simulink model "Pacemaker"  (R2020a)
settings: Solver=FixedStepAuto  StartTime=0.0  StopTime=10.0  FixedStep=1e-3  RelTol=1e-3  EnableMultiTasking=on
undefined symbols (not defined in the file): ATR_CMP_REF_PWM, ATR_GND_CTRL, ATR_PACE_CTRL, FRONTEND_CTRL, PACE_CHARGE_CTRL, PACE_GND_CTRL, PACING_REF_PWM, VENT_CMP_REF_PWM, VENT_GND_CTRL, VENT_PACE_CTRL, Z_ATR_CTRL, Z_VENT_CTRL
libraries: frdmk64flib x1
settings Model: ExtModeTrigDuration=5  Creator=Tim_G  LastModifiedBy=Tim_G
settings OptimizationCC: EnhancedBackFolding=on  PassReuseOutputArgsAs=Individual arguments  ZeroExternalMemoryAtStartup=off  ZeroInternalMemoryAtStartup=off  MaxStackSize=64  OptimizeBlockOrder=speed  DifferentSizesBufferReuse=on  OptimizationCustomize=off  EfficientTunableParamExpr=on
settings DebuggingCC: ParameterTunabilityLossMsg=error
settings HardwareCC: ProdBitPerPointer=32  ProdBitPerSizeT=32  ProdBitPerPtrDiffT=32  ProdLargestAtomicInteger=Long  ProdLargestAtomicFloat=Double  ProdWordSize=32  ProdHWDeviceType=ARM Compatible->ARM Cortex
settings SFSimCC: MATLABDynamicMemAlloc=off
settings RTWCC: SystemTargetFile=ert.tlc  HardwareBoard=NXP FRDM-K64F  TemplateMakefile=ert_default_tmf  Toolchain=GNU Tools for ARM Embedded Processors
settings CodeAppCC: ForceParamTrailComments=on  IgnoreCustomStorageClasses=off  OperatorAnnotations=on  SimulinkDataObjDesc=on  SFDataObjDesc=on  InsertBlockDesc=on

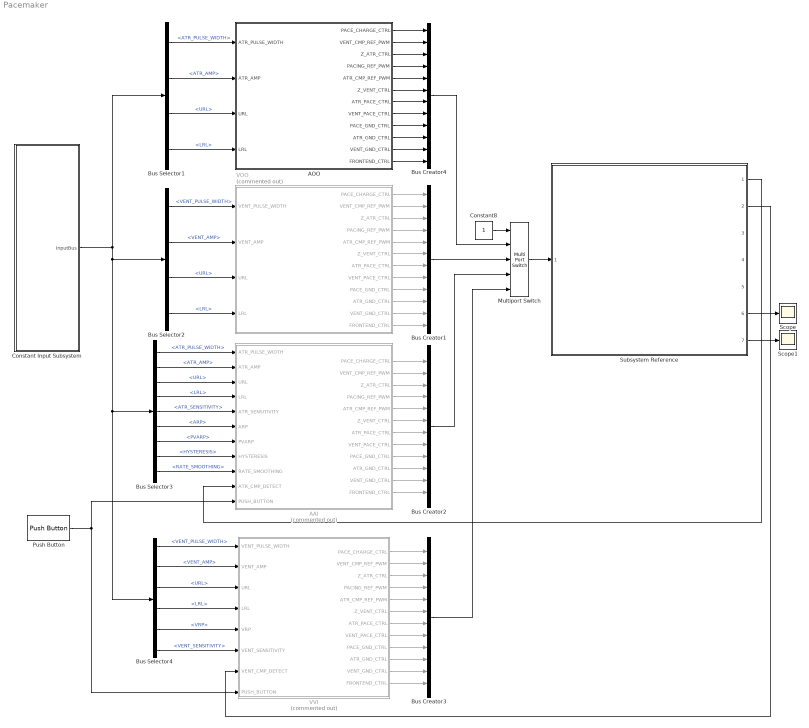
== system Pacemaker ==
  AAI : Stateflow chart  Commented=on  TreatAsAtomicUnit=on
      settings: PortSchema="{\"entries\":[{\"content\":{\"sides\":[{\"content\":{\"connectorIds\":[\"In1\",\"In2\",\"In3\",\"In4\",\"In6\",\"In5\",\"In8\",\"In9\",\"In10\",\"In7\",\"In11\"]},\"type\":\"ConnectorPlacement.EquallySpacedRectSide\",\"uuid\":\"15e17ad8-b4d5-4618-94ec-328f447b5375\"},{\"content\":{\"connectorIds\":[\"Out1\",\"Out2\",\"Out3\",\"Out4\",\"Out5\",\"Out6\",\"Out7\",\"Out8\",\"Out9\",\"Out10\",\"Out11\",\"Out12\"],\"side\":\"RIGHT\"},\"type\":\"ConnectorPlacement.EquallySpacedRectSide\",\"uuid\":\"1d62d0c4-23d6-4fac-9825-8cf7a4b74954\"},{\"content\":{\"connectorIds\":[],\"side\":\"TOP\"},\"type\":\"ConnectorPlacement.EquallySpacedRectSide\",\"uuid\":\"6d7cbaed-215f-4550-bcf7-2324ed1fe24a\"}]},\"type\":\"ConnectorPlacement.EquallySpacedConnector\",\"uuid\":\"41d78d22-c4a1-401b-9b90-f67359ce816a\"}],\"packageUris\":[\"http://schema.mathworks.com/mf0/Connector/19700101\"],\"version\":\"1.0\"}"
  AOO : Stateflow chart  TreatAsAtomicUnit=on
  Bus Creator{1..4} (4 alike) : BusCreator  Inputs=PACE_CHARGE_CTRL,VENT_CMP_REF_PWM,Z_ATR_CTRL,PACING_REF_PWM,ATR_CMP_REF_PWM,Z_VENT_CTRL,ATR_PACE_CTRL,VENT_PACE_CTRL,PACE_GND_CTRL,ATR_GND_CTRL,VENT_GND_CTRL,FRONTEND_CTRL
  Bus Selector1 : BusSelector  OutputSignals=ATR_PULSE_WIDTH,ATR_AMP,URL,LRL
  Bus Selector2 : BusSelector  OutputSignals=VENT_PULSE_WIDTH,VENT_AMP,URL,LRL
  Bus Selector3 : BusSelector  OutputSignals=ATR_PULSE_WIDTH,ATR_AMP,URL,LRL,ATR_SENSITIVITY,ARP,PVARP,HYSTERESIS,RATE_SMOOTHING
  Bus Selector4 : BusSelector  OutputSignals=VENT_PULSE_WIDTH,VENT_AMP,URL,LRL,VRP,VENT_SENSITIVITY
  Constant Input Subsystem : Subsystem
  Constant8 : Constant
  Multiport Switch : MultiPortSwitch  Inputs=4
  Push Button : frdmk64flib/Push Button  Whichswitch=SW2  SampleTime1=-1
  Scope : Scope
  Scope1 : Scope
  Subsystem Reference : Subsystem  ReferencedSubsystem=k64f_hardware_subsystem
  VOO : Stateflow chart  Commented=on  TreatAsAtomicUnit=on
  VVI : Stateflow chart  Commented=on  TreatAsAtomicUnit=on
  wires:
  AAI/3(Z_ATR_CTRL) -> Bus Creator2/3
  AAI/10(ATR_GND_CTRL) -> Bus Creator2/10
  AAI/11(VENT_GND_CTRL) -> Bus Creator2/11
  AAI/12(FRONTEND_CTRL) -> Bus Creator2/12
  Bus Creator2/1 -> Multiport Switch/4
  AAI/5(ATR_CMP_REF_PWM) -> Bus Creator2/5
  AAI/6(Z_VENT_CTRL) -> Bus Creator2/6
  AAI/4(PACING_REF_PWM) -> Bus Creator2/4
  AAI/9(PACE_GND_CTRL) -> Bus Creator2/9
  AAI/8(VENT_PACE_CTRL) -> Bus Creator2/8
  AAI/7(ATR_PACE_CTRL) -> Bus Creator2/7
  Bus Creator1/1 -> Multiport Switch/3
  Subsystem Reference/2 -> VVI/7(VENT_CMP_DETECT)
  AAI/1(PACE_CHARGE_CTRL) -> Bus Creator2/1
  Subsystem Reference/1 -> AAI/7(ATR_CMP_DETECT)
  Bus Creator4/1 -> Multiport Switch/2
  Constant8/1 -> Multiport Switch/1
  VVI/1(PACE_CHARGE_CTRL) -> Bus Creator3/1
  VVI/2(VENT_CMP_REF_PWM) -> Bus Creator3/2
  VVI/3(Z_ATR_CTRL) -> Bus Creator3/3
  VVI/4(PACING_REF_PWM) -> Bus Creator3/4
  VVI/6(Z_VENT_CTRL) -> Bus Creator3/6
  VVI/7(ATR_PACE_CTRL) -> Bus Creator3/7
  VVI/8(VENT_PACE_CTRL) -> Bus Creator3/8
  VVI/9(PACE_GND_CTRL) -> Bus Creator3/9
  VVI/10(ATR_GND_CTRL) -> Bus Creator3/10
  VVI/11(VENT_GND_CTRL) -> Bus Creator3/11
  VVI/12(FRONTEND_CTRL) -> Bus Creator3/12
  Bus Creator3/1 -> Multiport Switch/5
  Bus Selector1/1 -> AOO/1(ATR_PULSE_WIDTH)  "<ATR_PULSE_WIDTH>"
  Bus Selector1/2 -> AOO/2(ATR_AMP)  "<ATR_AMP>"
  Bus Selector1/3 -> AOO/3(URL)  "<URL>"
  Bus Selector1/4 -> AOO/4(LRL)  "<LRL>"
  Bus Selector3/1 -> AAI/1(ATR_PULSE_WIDTH)  "<ATR_PULSE_WIDTH>"
  Bus Selector3/2 -> AAI/2(ATR_AMP)  "<ATR_AMP>"
  Bus Selector3/3 -> AAI/3(URL)  "<URL>"
  Bus Selector3/4 -> AAI/4(LRL)  "<LRL>"
  Bus Selector3/7 -> AAI/8(PVARP)  "<PVARP>"
  Bus Selector3/8 -> AAI/9(HYSTERESIS)  "<HYSTERESIS>"
  Bus Selector3/9 -> AAI/10(RATE_SMOOTHING)  "<RATE_SMOOTHING>"
  Bus Selector3/5 -> AAI/6(ATR_SENSITIVITY)  "<ATR_SENSITIVITY>"
  Bus Selector3/6 -> AAI/5(ARP)  "<ARP>"
  Bus Selector4/1 -> VVI/1(VENT_PULSE_WIDTH)  "<VENT_PULSE_WIDTH>"
  Bus Selector4/2 -> VVI/2(VENT_AMP)  "<VENT_AMP>"
  Bus Selector4/3 -> VVI/3(URL)  "<URL>"
  Bus Selector4/4 -> VVI/4(LRL)  "<LRL>"
  Bus Selector4/5 -> VVI/5(VRP)  "<VRP>"
  Bus Selector4/6 -> VVI/6(VENT_SENSITIVITY)  "<VENT_SENSITIVITY>"
  Constant Input Subsystem/1(InputBus) -> Bus Selector2/1, Bus Selector4/1, Bus Selector3/1, Bus Selector1/1
  Push Button/1 -> VVI/8(PUSH_BUTTON), AAI/11(PUSH_BUTTON)
  AOO/1(PACE_CHARGE_CTRL) -> Bus Creator4/1
  AOO/2(VENT_CMP_REF_PWM) -> Bus Creator4/2
  AOO/3(Z_ATR_CTRL) -> Bus Creator4/3
  AOO/4(PACING_REF_PWM) -> Bus Creator4/4
  AOO/5(ATR_CMP_REF_PWM) -> Bus Creator4/5
  AOO/6(Z_VENT_CTRL) -> Bus Creator4/6
  AOO/7(ATR_PACE_CTRL) -> Bus Creator4/7
  AOO/8(VENT_PACE_CTRL) -> Bus Creator4/8
  AOO/9(PACE_GND_CTRL) -> Bus Creator4/9
  AOO/10(ATR_GND_CTRL) -> Bus Creator4/10
  AOO/11(VENT_GND_CTRL) -> Bus Creator4/11
  AOO/12(FRONTEND_CTRL) -> Bus Creator4/12
  VOO/1(PACE_CHARGE_CTRL) -> Bus Creator1/1
  VOO/2(VENT_CMP_REF_PWM) -> Bus Creator1/2
  VOO/3(Z_ATR_CTRL) -> Bus Creator1/3
  VOO/4(PACING_REF_PWM) -> Bus Creator1/4
  VOO/5(ATR_CMP_REF_PWM) -> Bus Creator1/5
  VOO/6(Z_VENT_CTRL) -> Bus Creator1/6
  VOO/7(ATR_PACE_CTRL) -> Bus Creator1/7
  VOO/8(VENT_PACE_CTRL) -> Bus Creator1/8
  VOO/9(PACE_GND_CTRL) -> Bus Creator1/9
  VOO/10(ATR_GND_CTRL) -> Bus Creator1/10
  VOO/11(VENT_GND_CTRL) -> Bus Creator1/11
  VOO/12(FRONTEND_CTRL) -> Bus Creator1/12
  AAI/2(VENT_CMP_REF_PWM) -> Bus Creator2/2
  VVI/5(ATR_CMP_REF_PWM) -> Bus Creator3/5
  Bus Selector2/1 -> VOO/1(VENT_PULSE_WIDTH)  "<VENT_PULSE_WIDTH>"
  Bus Selector2/2 -> VOO/2(VENT_AMP)  "<VENT_AMP>"
  Bus Selector2/3 -> VOO/3(URL)  "<URL>"
  Bus Selector2/4 -> VOO/4(LRL)  "<LRL>"
  Multiport Switch/1 -> Subsystem Reference/1
  Subsystem Reference/7 -> Scope1/1
  Subsystem Reference/6 -> Scope/1

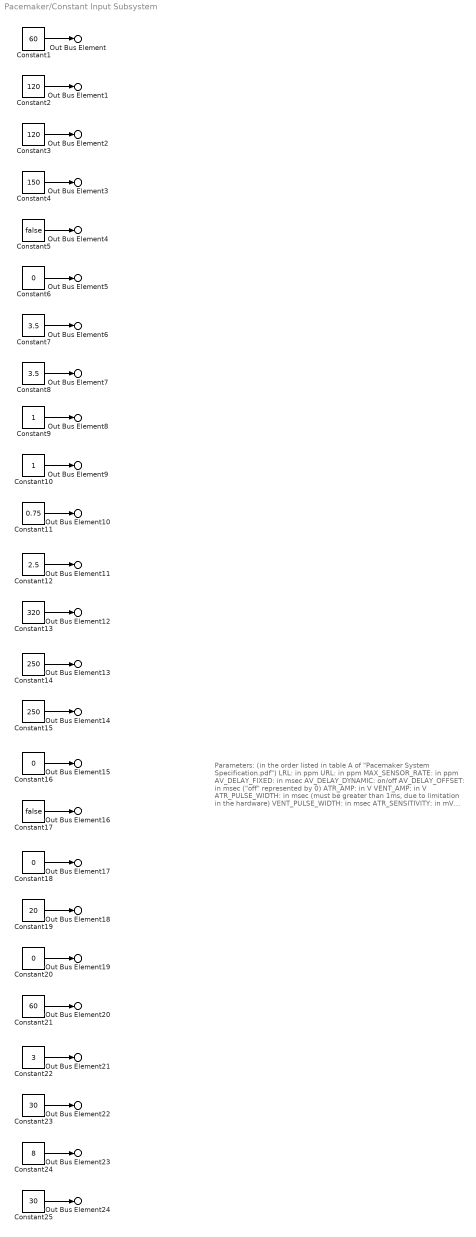
== system Pacemaker/Constant Input Subsystem ==
  note: Parameters:
      | (in the order listed in table A of "Pacemaker System Specification.pdf")
      | LRL: in ppm
      | URL: in ppm
      | MAX_SENSOR_RATE: in ppm
      | AV_DELAY_FIXED: in msec
      | AV_DELAY_DYNAMIC: on/off
      | AV_DELAY_OFFSET: in msec ("off" represented by 0)
      | ATR_AMP: in V
      | VENT_AMP: in V
      | ATR_PULSE_WIDTH: in msec (must be greater than 1ms, due to
      | limitation in the hardware)
      | VENT_PULSE_WIDTH: in msec
      | ATR_SENSITIVITY: in mV
      | VENT_SENSITIVITY: in mV
      | VRP: in msec
      | ARP: in msec
      | PVARP: in msec
      | PVARP_EXT: in msec ("off" represented by 0)
      | HYSTERESIS: off/same choices as LRL (represented by "on")
      | RATE_SMOOTHING: off represented by 0
      | ATR_DURATION: in cardiac cycles
      | ATR_FALLBACK_MODE
      | ATR_FALLBACK_TIME: in sec
      | ACT_THRESHOLD:
      | 0-V-Low
      | 1-Low
      | 2-Med-Low
      | 3-Med
      | 4-Med-High
      | 5-High
      | 6-V-High
      | REACTION_TIME: in sec
      | RESPONSE_FACTOR
      | RECOVERY_TIME: in sec
  Constant1 : Constant  Value=60
  Constant10 : Constant
  Constant11 : Constant  Value=0.75
  Constant12 : Constant  Value=2.5
  Constant13 : Constant  Value=320
  Constant14 : Constant  Value=250
  Constant15 : Constant  Value=250
  Constant{6,16,18,20} (4 alike) : Constant  Value=0
  Constant17 : Constant  Value=false
  Constant19 : Constant  Value=20
  Constant2 : Constant  Value=120
  Constant21 : Constant  Value=60
  Constant22 : Constant  Value=3
  Constant23 : Constant  Value=30
  Constant24 : Constant  Value=8
  Constant25 : Constant  Value=30
  Constant3 : Constant  Value=120
  Constant4 : Constant  Value=150
  Constant5 : Constant  Value=false
  Constant7 : Constant  Value=3.5
  Constant8 : Constant  Value=3.5
  Constant9 : Constant
  Out Bus Element : Outport  PortName=InputBus  Element=LRL
  Out Bus Element1 : Outport  PortName=InputBus  Element=URL
  Out Bus Element2 : Outport  PortName=InputBus  Element=MAX_SENSOR_RATE
  Out Bus Element3 : Outport  PortName=InputBus  Element=AV_DELAY_FIXED
  Out Bus Element4 : Outport  PortName=InputBus  Element=AV_DELAY_DYNAMIC
  Out Bus Element5 : Outport  PortName=InputBus  Element=AV_DELAY_OFFSET
  Out Bus Element6 : Outport  PortName=InputBus  Element=ATR_AMP
  Out Bus Element7 : Outport  PortName=InputBus  Element=VENT_AMP
  Out Bus Element8 : Outport  PortName=InputBus  Element=ATR_PULSE_WIDTH
  Out Bus Element9 : Outport  PortName=InputBus  Element=VENT_PULSE_WIDTH
  Out Bus Element10 : Outport  PortName=InputBus  Element=ATR_SENSITIVITY
  Out Bus Element11 : Outport  PortName=InputBus  Element=VENT_SENSITIVITY
  Out Bus Element12 : Outport  PortName=InputBus  Element=VRP
  Out Bus Element13 : Outport  PortName=InputBus  Element=ARP
  Out Bus Element14 : Outport  PortName=InputBus  Element=PVARP
  Out Bus Element15 : Outport  PortName=InputBus  Element=PVARP_EXT
  Out Bus Element16 : Outport  PortName=InputBus  Element=HYSTERESIS
  Out Bus Element17 : Outport  PortName=InputBus  Element=RATE_SMOOTHING
  Out Bus Element18 : Outport  PortName=InputBus  Element=ATR_DURATION
  Out Bus Element19 : Outport  PortName=InputBus  Element=ATR_FALLBACK_MODE
  Out Bus Element20 : Outport  PortName=InputBus  Element=ATR_FALLBACK_TIME
  Out Bus Element21 : Outport  PortName=InputBus  Element=ACT_THRESHOLD
  Out Bus Element22 : Outport  PortName=InputBus  Element=REACTION_TIME
  Out Bus Element23 : Outport  PortName=InputBus  Element=RESPONSE_FACTOR
  Out Bus Element24 : Outport  PortName=InputBus  Element=RECOVERY_TIME
  wires:
  Constant1/1 -> Out Bus Element/1
  Constant2/1 -> Out Bus Element1/1
  Constant4/1 -> Out Bus Element3/1
  Constant3/1 -> Out Bus Element2/1
  Constant5/1 -> Out Bus Element4/1
  Constant6/1 -> Out Bus Element5/1
  Constant8/1 -> Out Bus Element7/1
  Constant7/1 -> Out Bus Element6/1
  Constant10/1 -> Out Bus Element9/1
  Constant11/1 -> Out Bus Element10/1
  Constant9/1 -> Out Bus Element8/1
  Constant13/1 -> Out Bus Element12/1
  Constant12/1 -> Out Bus Element11/1
  Constant14/1 -> Out Bus Element13/1
  Constant15/1 -> Out Bus Element14/1
  Constant19/1 -> Out Bus Element18/1
  Constant18/1 -> Out Bus Element17/1
  Constant16/1 -> Out Bus Element15/1
  Constant17/1 -> Out Bus Element16/1
  Constant25/1 -> Out Bus Element24/1
  Constant24/1 -> Out Bus Element23/1
  Constant23/1 -> Out Bus Element22/1
  Constant22/1 -> Out Bus Element21/1
  Constant20/1 -> Out Bus Element19/1
  Constant21/1 -> Out Bus Element20/1

== stateflow chart Pacemaker/AOO ==
  note: Inputs:
      | ppm=LRL; (1/automatic interval)
      | ATR_AMP; (amplitude in V)
      | ATR_PULSE_WIDTH; (in msec)
  state Init
    entry:
    VENT_CMP_REF_PWM=100;
    ATR_CMP_REF_PWM=100;
    FRONTEND_CTRL=false;
  state Charging
    %% Charge C22
    entry:
    ATR_PACE_CTRL = false;
    VENT_PACE_CTRL = false;
    PACING_REF_PWM = ATR_AMP*20;
    %PACING_REF_PWM = ATR_AMP/5*100;
    PACE_CHARGE_CTRL = true;
    %% Discharge C21
    PACE_GND_CTRL = true;
    Z_ATR_CTRL = false;
    Z_VENT_CTRL = false;
    ATR_GND_CTRL = true;
    VENT_GND_CTRL = false;
  state Pacing
    entry:
    PACE_CHARGE_CTRL = false;
    PACE_GND_CTRL = true;
    ATR_PACE_CTRL = true;
    ATR_GND_CTRL = false;
    Z_ATR_CTRL = false;
    Z_VENT_CTRL =false;
    VENT_GND_CTRL = false;
    VENT_PACE_CTRL = false;
  (default) -> Init
  Charging -> Pacing : [after(60/LRL,sec)]
  Init -> Charging
  Pacing -> Charging : [after(ATR_PULSE_WIDTH,msec)]
  data: PACE_CHARGE_CTRL output boolean; VENT_CMP_REF_PWM output double; Z_ATR_CTRL output boolean; PACING_REF_PWM output double; ATR_CMP_REF_PWM output double; Z_VENT_CTRL output boolean; ATR_PACE_CTRL output boolean; VENT_PACE_CTRL output boolean; PACE_GND_CTRL output boolean; ATR_GND_CTRL output boolean; VENT_GND_CTRL output boolean; ATR_PULSE_WIDTH input double; ATR_AMP input double; URL input double; LRL input double; FRONTEND_CTRL output boolean

== stateflow chart Pacemaker/VOO ==
  note: Inputs:
      | ppm=LRL; (1/automatic interval)
      | VENT_AMP; (amplitude in V)
      | VENT_PULSE_WIDTH; (in msec)
  state Init
    entry:
    VENT_CMP_REF_PWM=100;
    ATR_CMP_REF_PWM=100;
    FRONTEND_CTRL=false;
  state Charging
    entry:
    %% Charge C22
    ATR_PACE_CTRL = false;
    VENT_PACE_CTRL = false;
    PACING_REF_PWM = VENT_AMP*20;
    %PACING_REF_PWM = VENT_AMP/5*100;
    PACE_CHARGE_CTRL = true;
    %% Discharge C21
    PACE_GND_CTRL = true;
    Z_ATR_CTRL = false;
    Z_VENT_CTRL = false;
    ATR_GND_CTRL = false;
    VENT_GND_CTRL = true;
  state Pacing
    entry:
    PACE_CHARGE_CTRL = false;
    PACE_GND_CTRL = true;
    ATR_PACE_CTRL = false;
    ATR_GND_CTRL = false;
    Z_ATR_CTRL = false;
    Z_VENT_CTRL = false;
    VENT_GND_CTRL = false;
    VENT_PACE_CTRL = true;
  (default) -> Init
  Charging -> Pacing : [after(60/LRL,sec)]
  Pacing -> Charging : [after(VENT_PULSE_WIDTH,msec)]
  Init -> Charging
  data: PACE_CHARGE_CTRL output boolean; VENT_CMP_REF_PWM output double; Z_ATR_CTRL output boolean; PACING_REF_PWM output double; ATR_CMP_REF_PWM output; Z_VENT_CTRL output boolean; ATR_PACE_CTRL output boolean; VENT_PACE_CTRL output boolean; PACE_GND_CTRL output boolean; ATR_GND_CTRL output boolean; VENT_GND_CTRL output boolean; VENT_PULSE_WIDTH input double; VENT_AMP input double; URL input double; LRL input double; FRONTEND_CTRL output boolean

== stateflow chart Pacemaker/VVI ==
  state REF_delay
  note: Inputs
      | VENT_SENSITIVITY; (sensing threshold in mV)
      | VRP; (ventricular refactory period, in msec)
      | ppm=LRL; (1/automatic interval)
      | VENT_AMP; (amplitude in V)
      | VENT_PULSE_WIDTH; (in msec)
      | VENT_CMP_DETECT (sensing signal from hardware)
  state Init
    entry:
    FRONTEND_CTRL = true;
    ATR_CMP_REF_PWM=100;
    VENT_CMP_REF_PWM =(51+VENT_SENSITIVITY)*1080/941;
    % see explanation for ...REF_PWM in section 2.3.4 of the Document
  state Charging
    entry:
    %% Charge C22
    ATR_PACE_CTRL = false;
    VENT_PACE_CTRL = false;
    PACING_REF_PWM = VENT_AMP*20;
    %PACING_REF_PWM = VENT_AMP/5*100;
    PACE_CHARGE_CTRL = true;
    %% Discharge C21
    PACE_GND_CTRL = true;
    Z_ATR_CTRL = false;
    Z_VENT_CTRL = false;
    ATR_GND_CTRL = false;
    VENT_GND_CTRL = true;
  state Pacing
    entry:
    PACE_CHARGE_CTRL = false;
    PACE_GND_CTRL = true;
    ATR_PACE_CTRL = false;
    ATR_GND_CTRL = false;
    Z_ATR_CTRL = false;
    Z_VENT_CTRL = false;
    VENT_GND_CTRL = false;
    VENT_PACE_CTRL = true;
  REF_delay -> Pacing [order 1] : [after(60000/LRL - VENT_PULSE_WIDTH - VRP, msec)]
  Charging -> REF_delay : [after(VRP,msec)]
  REF_delay -> Charging [order 2] : [VENT_CMP_DETECT == true || PUSH_BUTTON==true]
  (default) -> Init
  Pacing -> Charging : [after(VENT_PULSE_WIDTH,msec)]
  Init -> Charging
  data: PACE_CHARGE_CTRL output boolean; VENT_CMP_REF_PWM output double; Z_ATR_CTRL output boolean; PACING_REF_PWM output double; ATR_CMP_REF_PWM output double; VENT_PULSE_WIDTH input double; VENT_AMP input double; URL input double; LRL input double; VRP input double; VENT_SENSITIVITY input double; VENT_CMP_DETECT input boolean; Z_VENT_CTRL output boolean; ATR_PACE_CTRL output boolean; VENT_PACE_CTRL output boolean; PACE_GND_CTRL output boolean; ATR_GND_CTRL output boolean; VENT_GND_CTRL output boolean; FRONTEND_CTRL output boolean; PUSH_BUTTON input

== stateflow chart Pacemaker/AAI ==
  state REF_delay
  note: Inputs:
      | ATR_CMP_REF_PWM (duty cycle in %)
      | ARP; (atrial refactory period, in msec)
      | ppm= LRL; (1/automatic interval)
      | ATR_AMP (amplitude in V)
      | ATR_PULSE_WIDTH; (pulse width in msec)
      | ATR_CMP_DETECT; (sensing signal from hardware)
  state Charge
    entry:
    %% Charge C22
    ATR_PACE_CTRL = false;
    VENT_PACE_CTRL = false;
    PACING_REF_PWM = ATR_AMP*20;
    %PACING_REF_PWM = ATR_AMP/5*100;
    PACE_CHARGE_CTRL = true;
    %% Discharge C21
    PACE_GND_CTRL = true;
    Z_ATR_CTRL = false;
    Z_VENT_CTRL = false;
    ATR_GND_CTRL = true;
    VENT_GND_CTRL = false;
  state Pacing
    entry:
    PACE_CHARGE_CTRL = false;
    PACE_GND_CTRL = true;
    ATR_PACE_CTRL = true;
    ATR_GND_CTRL = false;
    Z_ATR_CTRL = false;
    Z_VENT_CTRL = false;
    VENT_GND_CTRL = false;
    VENT_PACE_CTRL = false;
  state Sensing
    entry:
    FRONTEND_CTRL = true;
    VENT_CMP_REF_PWM=100;
    ATR_CMP_REF_PWM = (58+ATR_SENSITIVITY)/0.82625;
    % see explanation for ...REF_PWM in section 2.3.4 of the Document
  REF_delay -> Pacing [order 1] : [after(60000/LRL - ATR_PULSE_WIDTH - ARP, msec)]
  Charge -> REF_delay : [after(ARP,msec)]
  REF_delay -> Charge [order 2] : [ATR_CMP_DETECT == true || PUSH_BUTTON==true]
  (default) -> Sensing
  Sensing -> Charge
  Pacing -> Charge : [after(ATR_PULSE_WIDTH,msec)]
  data: PACE_CHARGE_CTRL output boolean; VENT_CMP_REF_PWM output double; ATR_PULSE_WIDTH input double; ATR_AMP input double; URL input double; LRL input double; ARP input double; ATR_SENSITIVITY input double; ATR_CMP_DETECT input boolean; Z_ATR_CTRL output boolean; PACING_REF_PWM output double; ATR_CMP_REF_PWM output double; Z_VENT_CTRL output boolean; ATR_PACE_CTRL output boolean; VENT_PACE_CTRL output boolean; PACE_GND_CTRL output boolean; ATR_GND_CTRL output boolean; VENT_GND_CTRL output boolean; FRONTEND_CTRL output boolean; PVARP input double; HYSTERESIS input boolean; RATE_SMOOTHING input double; PUSH_BUTTON input
